simulink model "pi_SS_H2DF_2024a_GRU"  (R2024a)
settings: Solver=FixedStepAuto  StartTime=0.0  StopTime=inf  FixedStep=0.001  RelTol=1e-3  EnableMultiTasking=on
values from neighbouring files (symbols this model uses):
  C2C_NMPC = init_C2C_NMPC_H2DF(C2C_NMPC.expdata)    [run_SS_H2DF_control.m]
libraries: matrix_library x3, raspberrypiNetworklib x1
(part 1 of 3)
settings Model: SimulationMode=external  ExtModeTrigDuration=2  Creator=maxim  LastModifiedBy=winkler_a
settings SolverCC: PositivePriorityOrder=on
settings DataIOCC: LimitDataPoints=on  MaxDataPoints=10000  SaveOutput=off
settings OptimizationCC: EnhancedBackFolding=on  PassReuseOutputArgsAs=Individual arguments  ZeroExternalMemoryAtStartup=off  ZeroInternalMemoryAtStartup=off  MaxStackSize=64  OptimizeBlockOrder=speed  DifferentSizesBufferReuse=on  OptimizationCustomize=off  EfficientTunableParamExpr=on
settings DebuggingCC: ParameterTunabilityLossMsg=error
settings HardwareCC: ProdBitPerPointer=32  ProdBitPerSizeT=32  ProdBitPerPtrDiffT=32  ProdLargestAtomicInteger=Long  ProdLargestAtomicFloat=Double  ProdWordSize=32  ProdLongLongMode=on  ProdHWDeviceType=ARM Compatible->ARM Cortex
settings SFSimCC: SimUserSources=|
  | C2C_NMPC_model/C2C_NMPC_dyn_disc_phi_fun.c
  | C2C_NMPC_model/C2C_NMPC_dyn_disc_phi_fun_jac.c
  | C2C_NMPC_constraints/C2C_NMPC_constr_h_fun.c
  | C2C_NMPC_constraints/C2C_NMPC_constr_h_fun_jac_uxt_zt.c
  | C2C_NMPC_constraints/C2C_NMPC_constr_h_e_fun.c
  | C2C_NMPC_constraints/C2C_NMPC_constr_h_e_fun_jac_uxt_zt.c
  | acados_solver_sfunction_C2C_NMPC.c
  | acados_solver_C2C_NMPC.c
settings SFSimCC: SimUserIncludeDirs=|
  | /include
  | /include/acados_c
  | /include/blasfeo/include
  | /include/hpipm/include
  | /lib
  | /c_generated_code
settings SFSimCC: SimUserLibraries=|
  | libblasfeo.so
  | libacados.so
  | libhpipm.so
settings RTWCC: Description=Embedded Coder  SystemTargetFile=ert.tlc  HardwareBoard=Raspberry Pi  TemplateMakefile=ert_default_tmf  RTWUseSimCustomCode=on  Toolchain=GNU GCC Embedded Linux  BuildConfiguration=Faster Runs  GPUComputeCapability=3.5
settings RTWCC: CustomInclude=|
  | /include
  | /include/acados_c
  | /include/blasfeo/include
  | /include/hpipm/include
  | /lib
  | /c_generated_code
settings RTWCC: CustomSource=|
  | C2C_NMPC_model/C2C_NMPC_dyn_disc_phi_fun.c
  | C2C_NMPC_model/C2C_NMPC_dyn_disc_phi_fun_jac.c
  | C2C_NMPC_constraints/C2C_NMPC_constr_h_fun.c
  | C2C_NMPC_constraints/C2C_NMPC_constr_h_fun_jac_uxt_zt.c
  | C2C_NMPC_constraints/C2C_NMPC_constr_h_e_fun.c
  | C2C_NMPC_constraints/C2C_NMPC_constr_h_e_fun_jac_uxt_zt.c
  | acados_solver_sfunction_C2C_NMPC.c
  | acados_solver_C2C_NMPC.c
settings RTWCC: CustomLibrary=|
  | libblasfeo.so
  | libacados.so
  | libhpipm.so
settings CodeAppCC: ForceParamTrailComments=on  IgnoreCustomStorageClasses=off  OperatorAnnotations=on  SimulinkDataObjDesc=on  SFDataObjDesc=on  InsertBlockDesc=on
settings ERTTargetCC: SupportContinuousTime=on  SupportNonInlinedSFcns=on  SupportVariableSizeSignals=on  ExtMode=on  ExtModeStaticAlloc=on  ExtModeMaxTrigDuration=1000  ExtModeMexArgs='192.168.140.200' 0 17725

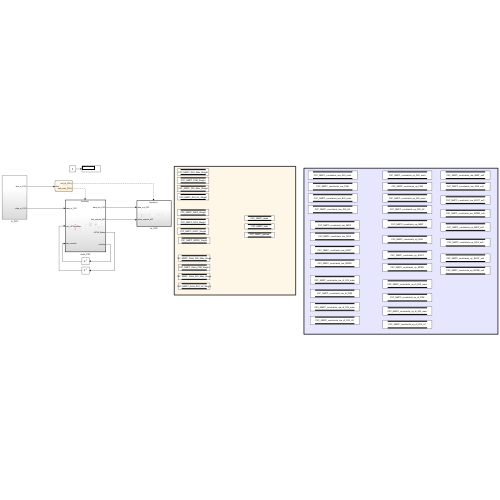
[thumbnail: Simulink's stored preview of the top-level diagram]
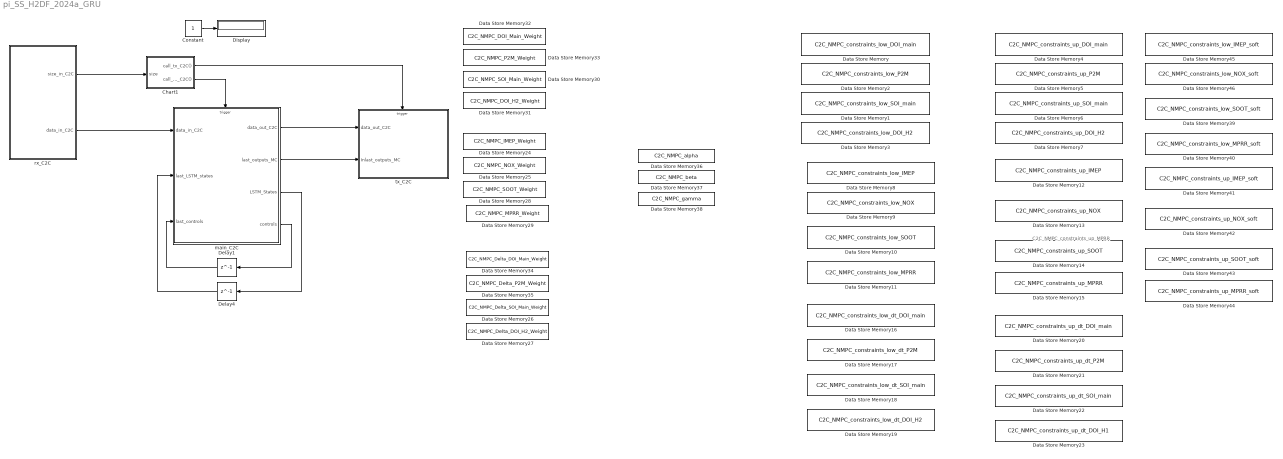
== system pi_SS_H2DF_2024a_GRU ==
  note: C2C_NMPC_constraints_up_MPRR
  Chart1 : Stateflow chart  TreatAsAtomicUnit=on
  Constant : Constant
  Data Store Memory : DataStoreMemory  DataStoreName=C2C_NMPC_constraints_low_DOI_main  WriteAfterWriteMsg=warning  ShowAdditionalParam=off
  Data Store Memory1 : DataStoreMemory  DataStoreName=C2C_NMPC_constraints_low_SOI_main  WriteAfterWriteMsg=warning  ShowAdditionalParam=off
  Data Store Memory10 : DataStoreMemory  DataStoreName=C2C_NMPC_constraints_low_SOOT  WriteAfterWriteMsg=warning  ShowAdditionalParam=off
  Data Store Memory11 : DataStoreMemory  DataStoreName=C2C_NMPC_constraints_low_MPRR  WriteAfterWriteMsg=warning  ShowAdditionalParam=off
  Data Store Memory12 : DataStoreMemory  DataStoreName=C2C_NMPC_constraints_up_IMEP  WriteAfterWriteMsg=warning  ShowAdditionalParam=off
  Data Store Memory13 : DataStoreMemory  DataStoreName=C2C_NMPC_constraints_up_NOX  WriteAfterWriteMsg=warning  ShowAdditionalParam=off
  Data Store Memory14 : DataStoreMemory  DataStoreName=C2C_NMPC_constraints_up_SOOT  WriteAfterWriteMsg=warning  ShowAdditionalParam=off
  Data Store Memory15 : DataStoreMemory  DataStoreName=C2C_NMPC_constraints_up_MPRR  WriteAfterWriteMsg=warning  ShowAdditionalParam=off
  Data Store Memory16 : DataStoreMemory  DataStoreName=C2C_NMPC_constraints_low_dt_DOI_main  WriteAfterWriteMsg=warning  ShowAdditionalParam=off
  Data Store Memory17 : DataStoreMemory  DataStoreName=C2C_NMPC_constraints_low_dt_P2M  WriteAfterWriteMsg=warning  ShowAdditionalParam=off
  Data Store Memory18 : DataStoreMemory  DataStoreName=C2C_NMPC_constraints_low_dt_SOI_main  WriteAfterWriteMsg=warning  ShowAdditionalParam=off
  Data Store Memory19 : DataStoreMemory  DataStoreName=C2C_NMPC_constraints_low_dt_DOI_H2  WriteAfterWriteMsg=warning  ShowAdditionalParam=off
  Data Store Memory2 : DataStoreMemory  DataStoreName=C2C_NMPC_constraints_low_P2M  WriteAfterWriteMsg=warning  ShowAdditionalParam=off
  Data Store Memory20 : DataStoreMemory  DataStoreName=C2C_NMPC_constraints_up_dt_DOI_main  WriteAfterWriteMsg=warning  ShowAdditionalParam=off
  Data Store Memory21 : DataStoreMemory  DataStoreName=C2C_NMPC_constraints_up_dt_P2M  WriteAfterWriteMsg=warning  ShowAdditionalParam=off
  Data Store Memory22 : DataStoreMemory  DataStoreName=C2C_NMPC_constraints_up_dt_SOI_main  WriteAfterWriteMsg=warning  ShowAdditionalParam=off
  Data Store Memory23 : DataStoreMemory  DataStoreName=C2C_NMPC_constraints_up_dt_DOI_H1  WriteAfterWriteMsg=warning  ShowAdditionalParam=off
  Data Store Memory24 : DataStoreMemory  DataStoreName=C2C_NMPC_IMEP_Weight  WriteAfterWriteMsg=warning  ShowAdditionalParam=off
  Data Store Memory25 : DataStoreMemory  DataStoreName=C2C_NMPC_NOX_Weight  WriteAfterWriteMsg=warning  ShowAdditionalParam=off
  Data Store Memory26 : DataStoreMemory  DataStoreName=C2C_NMPC_Delta_SOI_Main_Weight  WriteAfterWriteMsg=warning  ShowAdditionalParam=off
  Data Store Memory27 : DataStoreMemory  DataStoreName=C2C_NMPC_Delta_DOI_H2_Weight  WriteAfterWriteMsg=warning  ShowAdditionalParam=off
  Data Store Memory28 : DataStoreMemory  DataStoreName=C2C_NMPC_SOOT_Weight  WriteAfterWriteMsg=warning  ShowAdditionalParam=off
  Data Store Memory29 : DataStoreMemory  DataStoreName=C2C_NMPC_MPRR_Weight  WriteAfterWriteMsg=warning  ShowAdditionalParam=off
  Data Store Memory3 : DataStoreMemory  DataStoreName=C2C_NMPC_constraints_low_DOI_H2  WriteAfterWriteMsg=warning  ShowAdditionalParam=off
  Data Store Memory30 : DataStoreMemory  DataStoreName=C2C_NMPC_SOI_Main_Weight  WriteAfterWriteMsg=warning  ShowAdditionalParam=off
  Data Store Memory31 : DataStoreMemory  DataStoreName=C2C_NMPC_DOI_H2_Weight  WriteAfterWriteMsg=warning  ShowAdditionalParam=off
  Data Store Memory32 : DataStoreMemory  DataStoreName=C2C_NMPC_DOI_Main_Weight  WriteAfterWriteMsg=warning  ShowAdditionalParam=off
  Data Store Memory33 : DataStoreMemory  DataStoreName=C2C_NMPC_P2M_Weight  WriteAfterWriteMsg=warning  ShowAdditionalParam=off
  Data Store Memory34 : DataStoreMemory  DataStoreName=C2C_NMPC_Delta_DOI_Main_Weight  WriteAfterWriteMsg=warning  ShowAdditionalParam=off
  Data Store Memory35 : DataStoreMemory  DataStoreName=C2C_NMPC_Delta_P2M_Weight  WriteAfterWriteMsg=warning  ShowAdditionalParam=off
  Data Store Memory36 : DataStoreMemory  DataStoreName=C2C_NMPC_alpha  WriteAfterWriteMsg=warning  ShowAdditionalParam=off
  Data Store Memory37 : DataStoreMemory  DataStoreName=C2C_NMPC_beta  WriteAfterWriteMsg=warning  ShowAdditionalParam=off
  Data Store Memory38 : DataStoreMemory  DataStoreName=C2C_NMPC_gamma  WriteAfterWriteMsg=warning  ShowAdditionalParam=off
  Data Store Memory39 : DataStoreMemory  DataStoreName=C2C_NMPC_constraints_low_SOOT_soft  WriteAfterWriteMsg=warning  ShowAdditionalParam=off
  Data Store Memory4 : DataStoreMemory  DataStoreName=C2C_NMPC_constraints_up_DOI_main  WriteAfterWriteMsg=warning  ShowAdditionalParam=off
  Data Store Memory40 : DataStoreMemory  DataStoreName=C2C_NMPC_constraints_low_MPRR_soft  WriteAfterWriteMsg=warning  ShowAdditionalParam=off
  Data Store Memory41 : DataStoreMemory  DataStoreName=C2C_NMPC_constraints_up_IMEP_soft  WriteAfterWriteMsg=warning  ShowAdditionalParam=off
  Data Store Memory42 : DataStoreMemory  DataStoreName=C2C_NMPC_constraints_up_NOX_soft  WriteAfterWriteMsg=warning  ShowAdditionalParam=off
  Data Store Memory43 : DataStoreMemory  DataStoreName=C2C_NMPC_constraints_up_SOOT_soft  WriteAfterWriteMsg=warning  ShowAdditionalParam=off
  Data Store Memory44 : DataStoreMemory  DataStoreName=C2C_NMPC_constraints_up_MPRR_soft  WriteAfterWriteMsg=warning  ShowAdditionalParam=off
  Data Store Memory45 : DataStoreMemory  DataStoreName=C2C_NMPC_constraints_low_IMEP_soft  WriteAfterWriteMsg=warning  ShowAdditionalParam=off
  Data Store Memory46 : DataStoreMemory  DataStoreName=C2C_NMPC_constraints_low_NOX_soft  WriteAfterWriteMsg=warning  ShowAdditionalParam=off
  Data Store Memory5 : DataStoreMemory  DataStoreName=C2C_NMPC_constraints_up_P2M  WriteAfterWriteMsg=warning  ShowAdditionalParam=off
  Data Store Memory6 : DataStoreMemory  DataStoreName=C2C_NMPC_constraints_up_SOI_main  WriteAfterWriteMsg=warning  ShowAdditionalParam=off
  Data Store Memory7 : DataStoreMemory  DataStoreName=C2C_NMPC_constraints_up_DOI_H2  WriteAfterWriteMsg=warning  ShowAdditionalParam=off
  Data Store Memory8 : DataStoreMemory  DataStoreName=C2C_NMPC_constraints_low_IMEP  WriteAfterWriteMsg=warning  ShowAdditionalParam=off
  Data Store Memory9 : DataStoreMemory  DataStoreName=C2C_NMPC_constraints_low_NOX  WriteAfterWriteMsg=warning  ShowAdditionalParam=off
  Delay1 : Delay  DelayLength=1  InitialCondition=C2C_NMPC.x0([(C2C_NMPC.Dims.n_LSTM_states + 1):(C2C_NMPC.Dims.n_LSTM_states + C2C_NMPC.Dims.n_controls)])
  Delay4 : Delay  DelayLength=1  InitialCondition=C2C_NMPC.x0(1:C2C_NMPC.Dims.n_LSTM_states)
  Display : Display
  main_C2C : Subsystem
  rx_C2C : Subsystem
  tx_C2C : Subsystem
  wires:
  rx_C2C/1(size_in_C2C) -> Chart1/1(size)
  rx_C2C/2(data_in_C2C) -> main_C2C/1(data_in_C2C)
  Chart1/2(call_main_C2C()) -> main_C2C/Trigger
  Constant/1 -> Display/1
  main_C2C/1(data_out_C2C) -> tx_C2C/1(data_out_C2C)
  main_C2C/2(last_outputs_MC) -> tx_C2C/2(Inlast_outputs_MC)
  Chart1/1(call_tx_C2C()) -> tx_C2C/Trigger
  main_C2C/4(controls) -> Delay1/1
  main_C2C/3(LSTM_States) -> Delay4/1
  Delay1/1 -> main_C2C/3(last_controls)
  Delay4/1 -> main_C2C/2(last_LSTM_states)

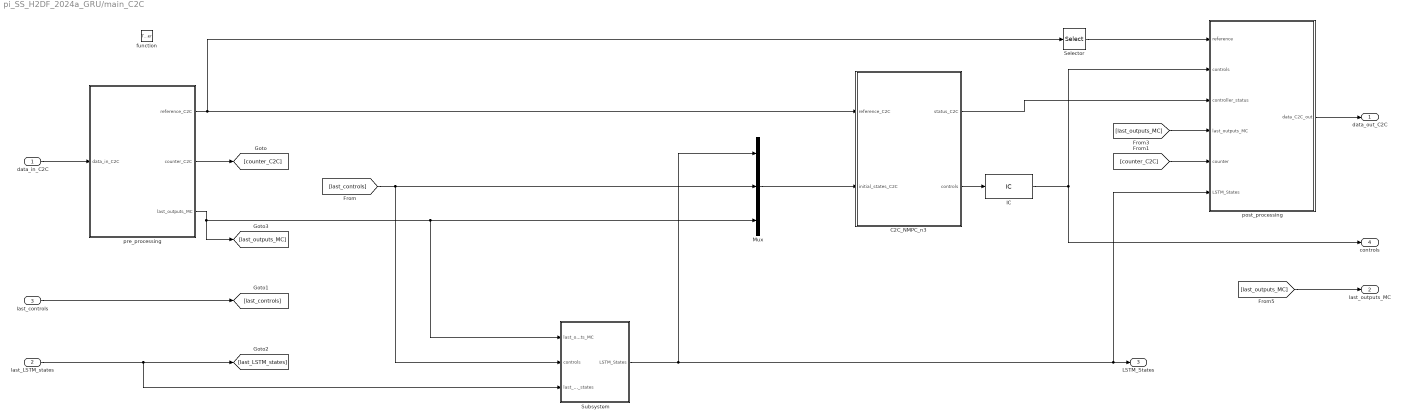
== system pi_SS_H2DF_2024a_GRU/main_C2C ==
  data_in_C2C : Inport
  last_LSTM_states : Inport  Port=2
  last_controls : Inport  Port=3
  function : TriggerPort  TriggerType=function-call  VariantControl=(inherit)
  C2C_NMPC_n3 : Subsystem  VariantControl=C2C_NMPC_n3
  IC : InitialCondition  Value=C2C_NMPC.x0([(C2C_NMPC.Dims.n_LSTM_states + 1):(C2C_NMPC.Dims.n_LSTM_states + C2C_NMPC.Dims.n_controls)])
  Mux : Mux  Inputs=3
  Selector : Selector  InputPortWidth=C2C_NMPC.Dims.n_cost*3  IndexOptions=Index vector (dialog)  Indices=1:C2C_NMPC.Dims.n_cost  OutputSizes=1
  Subsystem : Subsystem
  post_processing : Subsystem
  pre_processing : Subsystem
  data_out_C2C : Outport
  last_outputs_MC : Outport  Port=2
  LSTM_States : Outport  Port=3
  controls : Outport  Port=4
  wires:
  IC/1 -> post_processing/2(controls), controls/1
  C2C_NMPC_n3/2(controls) -> IC/1
  last_LSTM_states/1 -> Subsystem/3(last_LSTM_states), [last_LSTM_states]
  data_in_C2C/1 -> pre_processing/1(data_in_C2C)
  Subsystem/1(LSTM_States) -> Mux/1, post_processing/6(LSTM_States), LSTM_States/1
  Mux/1 -> C2C_NMPC_n3/2(initial_states_C2C)
  pre_processing/2(counter_C2C) -> [counter_C2C]
  pre_processing/3(last_outputs_MC) -> Subsystem/1(last_outputs_MC), Mux/3, [last_outputs_MC]
  [last_outputs_MC] -> last_outputs_MC/1
  [counter_C2C] -> post_processing/5(counter)
  Selector/1 -> post_processing/1(reference)
  last_controls/1 -> [last_controls]
  [last_outputs_MC] -> post_processing/4(last_outputs_MC)
  [last_controls] -> Subsystem/2(controls), Mux/2
  C2C_NMPC_n3/1(status_C2C) -> post_processing/3(controller_status)
  post_processing/1(data_C2C_out) -> data_out_C2C/1
  pre_processing/1(reference_C2C) -> C2C_NMPC_n3/1(reference_C2C), Selector/1

== system pi_SS_H2DF_2024a_GRU/rx_C2C ==
  Data Type Conversion : DataTypeConversion  OutDataTypeStr=double  SaturateOnIntegerOverflow=off  RndMeth=Floor
  Receive : Subsystem
  Terminator : Terminator
  UDP Receive1 : raspberrypiNetworklib/UDP Receive  localURL='0.0.0.0'  localPort=42785  remoteURL='0.0.0.0'  remotePort=-1  recvBufferSize=8192  signalDatatype=uint32  dims=56  isVarSize=off  showBlockingTime=off  blockingTime=0  sampletime=0.001  blockPlatform=Raspberry Pi
  size_in_C2C : Outport
  data_in_C2C : Outport  Port=2
  wires:
  UDP Receive1/2 -> size_in_C2C/1
  UDP Receive1/1 -> Data Type Conversion/1
  Receive/1(udp_outputs) -> data_in_C2C/1
  Data Type Conversion/1 -> Receive/1(udp_data_in)
  Receive/2(controller_mode) -> Terminator/1

== system pi_SS_H2DF_2024a_GRU/tx_C2C ==
  note: [1:4,13,99:134,14,15,16,17,71:74]
  data_out_C2C : Inport
  Inlast_outputs_MC : Inport  Port=2
  function : TriggerPort  TriggerType=function-call  VariantControl=(inherit)
  Data Type Conversion : DataTypeConversion  OutDataTypeStr=uint32  SaturateOnIntegerOverflow=off  RndMeth=Floor
  Selector : Selector  IndexOptions=Index vector (dialog)  Indices=[1:4,13,115:142,14,15,16,17,95:98]  OutputSizes=1
  Subsystem : Subsystem
  Terminator : Terminator
  UDP Send1 : S-Function  AncestorBlock=raspberrypiNetworklib/UDP Send  InitFcn=|  FunctionName=sdspToNetwork  Parameters=localURL, localPortSource, localPort, remoteURL, remotePort, 8192, separateLengthPort, []  SFunctionDeploymentMode=off  EnableBusSupport=off  mask(UDP Send){remoteURL='192.168.140.159', remotePort=42784, localURL='0.0.0.0', localPortSource=Specify via dialog, localPort=42784, sampletime=-1, blockPlatform=Raspberry Pi, separateLengthPort=0}
      | realtime.internal.validateLinuxBlock(get_param(gcbh, 'blockPlatform'), gcbh);
      | realtime.internal.registerLinuxBlock(gcb);
      mask prompts: remoteURL "Remote IP address ('255.255.255.255' for broadcast):"; remotePort "Remote IP port:"; localURL "Local IP address:"; localPortSource "Local IP port source:"; localPort "Local IP port:"; blockPlatform "Block Platform"; separateLengthPort "Use a separate length port"
      mask help: Sends UDP packets to another UDP host on an Internet network. Set Remote IP address parameter to the IP address of the receiving UDP host. Set the Remote IP port parameter to the port number used by the receiving UDP host.
      mask Help: eval('realtime.helpView(get_param(gcb, ''blockPlatform''), [realtime.internal.getHelpLinkPrefix(gcb) ''libudpsend''])');
      mask TypeOptions localPortSource: Automatically determine | Specify via dialog
      mask Callback localPortSource:
      | mask_vis = get_param(gcbh, 'MaskVisibilities');
      | if strcmp(get_param(gcbh,'localPortSource'),'Specify via dialog')
      |     mask_vis{5} = 'on';
      | else
      |     mask_vis{5} = 'off';
      | end
      | set_param(gcbh, 'MaskVisibilities', mask_vis);
      | clear('mask_vis');
      mask Display:
      | %fprintf('UDP Send');
      | color('blue');
      | [data, map]=imread('ethernet2_bw.gif');pic=ind2rgb(data,map);image(pic,[0.32 0.25 0.40 0.45]);
      | platform = realtime.internal.getBlockDisplayText(gcb);
      | text(0.99, 0.9, platform, 'horizontalalignment', 'right');
  wires:
  data_out_C2C/1 -> Selector/1
  Data Type Conversion/1 -> UDP Send1/1
  Selector/1 -> Subsystem/1(In1)
  Subsystem/1(Out1) -> Data Type Conversion/1
  Inlast_outputs_MC/1 -> Terminator/1

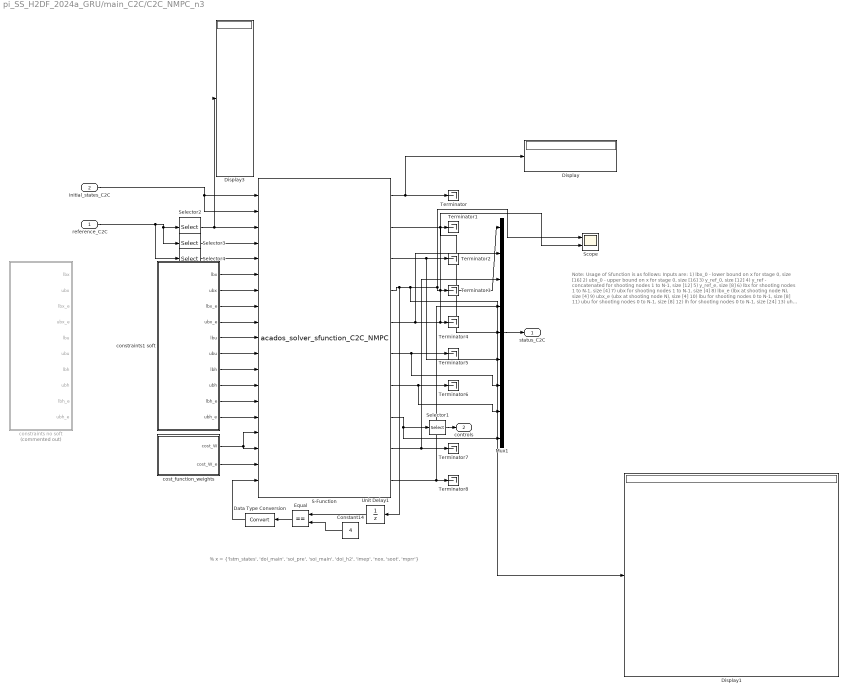
== system pi_SS_H2DF_2024a_GRU/main_C2C/C2C_NMPC_n3 ==
  note: Note: Usage of Sfunction is as follows:
      | Inputs are:
      | 1) lbx_0 - lower bound on x for stage 0, size [16]
      | 2) ubx_0 - upper bound on x for stage 0, size [16]
      | 3) y_ref_0, size [12]
      | 4) y_ref - concatenated for shooting nodes 1 to N-1, size [12]
      | 5) y_ref_e, size [8]
      | 6) lbx for shooting nodes 1 to N-1, size [4]
      | 7) ubx for shooting nodes 1 to N-1, size [4]
      | 8) lbx_e (lbx at shooting node N), size [4]
      | 9) ubx_e (ubx at shooting node N), size [4]
      | 10) lbu for shooting nodes 0 to N-1, size [8]
      | 11) ubu for shooting nodes 0 to N-1, size [8]
      | 12) lh for shooting nodes 0 to N-1, size [24]
      | 13) uh for shooting nodes 0 to N-1, size [24]
      | 14) lh_e, size [8]
      | 15) uh_e, size [8]
      | 16) cost_W_0 in column-major format, size [144]
      | 17) cost_W in column-major format, that is set for all intermediate shooting nodes: 1 to N-1, size [144]
      | 18) cost_W_e in column-major format, size [64]
      | 19) reset_solver determines if iterate is set to all zeros before other initializations (x_init, u_init) are set and before solver is called, size [1]
      |
      | Outputs are:
      | 1) u0, control input at node 0, size [4]
      | 2) utraj, control input concatenated for nodes 0 to N-1, size [8]
      | 3) xtraj, state concatenated for nodes 0 to N, size [48]
      | 4) acados solver status (0 = SUCCESS)
      | 5) cost function value
      | 6) KKT residual
      | 7) KKT residuals, size [4] (stat, eq, ineq, comp)
      | 8) x1, state at node 1
      | 9) CPU time
      | 10) SQP iterations
  note: % x = {'lstm_states', 'doi_main', 'soi_pre', 'soi_main', 'doi_h2', 'imep', 'nox, 'soot', 'mprr'}
  reference_C2C : Inport
  initial_states_C2C : Inport  Port=2
  Constant14 : Constant  Value=4
  Data Type Conversion : DataTypeConversion  SaturateOnIntegerOverflow=off  RndMeth=Floor
  Display : Display
  Display1 : Display
  Display3 : Display
  Equal : RelationalOperator  Operator===  OutDataTypeStr=boolean  RndMeth=Simplest  InputSameDT=off
  Mux1 : Mux  Inputs=9
  S-Function : S-Function  FunctionName=acados_solver_sfunction_C2C_NMPC  SFunctionDeploymentMode=off  EnableBusSupport=off
  Scope : Scope  NumInputPorts=2
  Selector1 : Selector  IndexOptions=Index vector (dialog)  Indices=[(C2C_NMPC.Dims.n_LSTM_states + 1):(C2C_NMPC.Dims.n_LSTM_states + C2C_NMPC.Dims.n_controls)]  OutputSizes=1
  Selector2 : Selector  IndexOptions=Index vector (dialog)  Indices=[1:(C2C_NMPC.Dims.n_cost)]  OutputSizes=1
  Selector3 : Selector  IndexOptions=Index vector (dialog)  Indices=[ (C2C_NMPC.Dims.n_cost + 1) : (C2C_NMPC.Dims.n_cost * 3) ]  OutputSizes=1
  Selector4 : Selector  IndexOptions=Index vector (dialog)  Indices=[ (C2C_NMPC.Dims.n_cost * 2 + 1) : (C2C_NMPC.Dims.n_cost * 2 + C2C_NMPC.Dims.n_controls + C2C_NMPC.Dims.n_outputs ) ]  OutputSizes=1
  Terminator{,1..8} (9 alike) : Terminator
  Unit Delay1 : UnitDelay  SampleTime=-1  HasFrameUpgradeWarning=on
  constraints no soft : Subsystem  Commented=on
  "constraints1 soft " : Subsystem
  cost_function_weights : Subsystem
  status_C2C : Outport
  controls : Outport  Port=2
  wires:
  "constraints1 soft "/5(lbu) -> S-Function/10
  "constraints1 soft "/6(ubu) -> S-Function/11
  "constraints1 soft "/7(lbh) -> S-Function/12
  "constraints1 soft "/8(ubh) -> S-Function/13
  "constraints1 soft "/9(lbh_e) -> S-Function/14
  "constraints1 soft "/10(ubh_e) -> S-Function/15
  cost_function_weights/1(cost_W) -> S-Function/16, S-Function/17
  Data Type Conversion/1 -> S-Function/19
  cost_function_weights/2(cost_W_e) -> S-Function/18
  "constraints1 soft "/1(lbx) -> S-Function/6
  "constraints1 soft "/2(ubx) -> S-Function/7
  "constraints1 soft "/3(lbx_e) -> S-Function/8
  "constraints1 soft "/4(ubx_e) -> S-Function/9
  S-Function/5 -> Mux1/2, Terminator4/1, Scope/2
  Equal/1 -> Data Type Conversion/1
  Unit Delay1/1 -> Equal/1
  Constant14/1 -> Equal/2
  Mux1/1 -> status_C2C/1
  Selector1/1 -> controls/1
  Selector4/1 -> S-Function/5
  reference_C2C/1 -> Selector4/1, Selector3/1, Selector2/1
  initial_states_C2C/1 -> S-Function/1, S-Function/2
  S-Function/10 -> Terminator8/1, Mux1/4
  S-Function/9 -> Terminator7/1, Mux1/3
  S-Function/7 -> Terminator6/1, Mux1/8
  S-Function/6 -> Terminator5/1, Mux1/7
  S-Function/8 -> Selector1/1, Mux1/9
  S-Function/4 -> Unit Delay1/1, Scope/1, Mux1/1, Terminator3/1, Display1/1
  S-Function/3 -> Terminator2/1, Mux1/6
  S-Function/2 -> Terminator1/1, Mux1/5
  S-Function/1 -> Display/1, Terminator/1
  Selector2/1 -> Display3/1, S-Function/3
  Selector3/1 -> S-Function/4

== system pi_SS_H2DF_2024a_GRU/main_C2C/Subsystem ==
  last_outputs_MC : Inport
  controls : Inport  Port=2
  last_LSTM_states : Inport  Port=3
  dyn_H2DF_state_augmentation : Subsystem
  LSTM_States : Outport
  wires:
  dyn_H2DF_state_augmentation/1(LSTM_states) -> LSTM_States/1
  controls/1 -> dyn_H2DF_state_augmentation/2(controls)
  last_outputs_MC/1 -> dyn_H2DF_state_augmentation/1(last_outputs_MC)
  last_LSTM_states/1 -> dyn_H2DF_state_augmentation/3(last_LSTM_states)

== system pi_SS_H2DF_2024a_GRU/main_C2C/post_processing ==
  reference : Inport
  controls : Inport  Port=2
  controller_status : Inport  Port=3
  last_outputs_MC : Inport  Port=4
  counter : Inport  Port=5
  LSTM_States : Inport  Port=6
  " denormalizing reference" : Subsystem
  Demux1 : Demux
  Demux2 : Demux
  Demux3 : Demux
  Display : Display  Commented=on
  Mux{8..11} (4 alike) : Mux  Inputs=2
  Mux4 : Mux
  Mux5 : Mux  Inputs=6
  Mux6 : Mux
  Selector5 : Selector  IndexOptions=Index vector (dialog)  Indices=[(C2C_NMPC.Dims.n_controls + 1 ):(C2C_NMPC.Dims.n_cost - C2C_NMPC.Dims.n_controls)]  OutputSizes=1
  Subsystem1 : Subsystem
  denormalizing physical controls and outputs : Subsystem
  data_C2C_out : Outport
  wires:
  Demux3/1 -> " denormalizing reference"/1(IMEP_norm)
  Demux3/2 -> " denormalizing reference"/2(NOX_norm)
  Demux3/4 -> " denormalizing reference"/4(MPRR_norm)
  Demux3/3 -> " denormalizing reference"/3(soot_norm)
  reference/1 -> Selector5/1
  Selector5/1 -> Demux3/1
  controls/1 -> Demux2/1
  Demux1/1 -> denormalizing physical controls and outputs/1(IMEP_norm)
  Demux1/2 -> denormalizing physical controls and outputs/2(NOX_norm)
  Demux1/3 -> denormalizing physical controls and outputs/3(soot_norm)
  Demux1/4 -> denormalizing physical controls and outputs/4(MPRR_norm)
  Demux2/1 -> denormalizing physical controls and outputs/5(DOI_main_norm)
  Demux2/2 -> denormalizing physical controls and outputs/6(SOI_pre_norm)
  Demux2/3 -> denormalizing physical controls and outputs/7(SOI_main_norm)
  denormalizing physical controls and outputs/5(DOI_main) -> Mux6/1
  denormalizing physical controls and outputs/6(SOI_pre) -> Mux6/2
  denormalizing physical controls and outputs/7(SOI_main) -> Mux6/3
  " denormalizing reference"/1(IMEP) -> Mux11/1
  " denormalizing reference"/2(NOX) -> Mux9/1
  " denormalizing reference"/3(soot) -> Mux8/1
  " denormalizing reference"/4(MPRR) -> Mux10/1
  controller_status/1 -> Mux5/4, Subsystem1/1(controller_ status)
  Mux5/1 -> data_C2C_out/1
  Mux11/1 -> Mux4/1
  Mux8/1 -> Mux4/3
  Mux10/1 -> Mux4/4
  denormalizing physical controls and outputs/1(IMEP) -> Mux11/2
  denormalizing physical controls and outputs/2(NOX) -> Mux9/2
  denormalizing physical controls and outputs/3(soot) -> Mux8/2
  denormalizing physical controls and outputs/4(MPRR) -> Mux10/2
  Mux4/1 -> Mux5/2
  counter/1 -> Mux5/3
  Mux6/1 -> Display/1, Mux5/1
  Demux2/4 -> denormalizing physical controls and outputs/8(DOI_H2_norm)
  denormalizing physical controls and outputs/8(DOI_H2) -> Mux6/4
  Mux9/1 -> Mux4/2
  LSTM_States/1 -> Mux5/5
  last_outputs_MC/1 -> Subsystem1/2(Last_Output_MC), Demux1/1
  Subsystem1/1(Out1) -> Mux5/6

== system pi_SS_H2DF_2024a_GRU/main_C2C/pre_processing ==
  data_in_C2C : Inport
  Selector : Selector  IndexOptions=Index vector (dialog)  Indices=[6]  OutputSizes=1
  normalize_last_outputs_MC : Subsystem
  normalize_reference_C2C : Subsystem
  reference_C2C : Outport  VectorParamsAs1DForOutWhenUnconnected=off
  counter_C2C : Outport  Port=2  VectorParamsAs1DForOutWhenUnconnected=off
  last_outputs_MC : Outport  Port=3  VectorParamsAs1DForOutWhenUnconnected=off
  wires:
  normalize_reference_C2C/1(reference_C2C) -> reference_C2C/1
  data_in_C2C/1 -> Selector/1, normalize_last_outputs_MC/1(data_in), normalize_reference_C2C/1(data_in)
  normalize_last_outputs_MC/1(last_outputs_MC) -> last_outputs_MC/1
  Selector/1 -> counter_C2C/1

== system pi_SS_H2DF_2024a_GRU/rx_C2C/Receive ==
  note: block for horizon of 3 from engine
  udp_data_in : Inport
  conversion_n3 : Subsystem
  udp_outputs : Outport
  controller_mode : Outport  Port=2
  wires:
  udp_data_in/1 -> conversion_n3/1(udp_data_in)
  conversion_n3/1(udp_outputs) -> udp_outputs/1
  conversion_n3/2(controller_mode) -> controller_mode/1

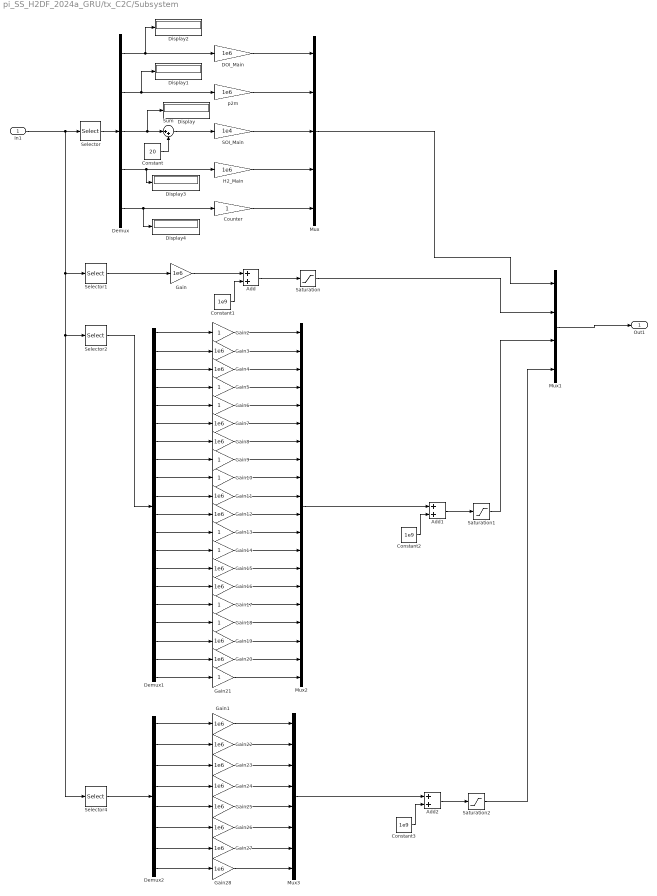
== system pi_SS_H2DF_2024a_GRU/tx_C2C/Subsystem ==
  In1 : Inport
  Add : Sum
  Add1 : Sum
  Add2 : Sum
  Constant : Constant  Value=20
  Constant1 : Constant  Value=1e9
  Constant2 : Constant  Value=1e9
  Constant3 : Constant  Value=1e9
  Counter : Gain
  DOI_Main : Gain  Gain=1e6
  Demux : Demux  Outputs=5
  Demux1 : Demux  Outputs=20
  Demux2 : Demux  Outputs=8
  Display{,1..4} (5 alike) : Display
  Gain{,1,3..4,7..8,11..12,15..16,19..20,22..28} (19 alike) : Gain  Gain=1e6
  Gain{2,5..6,9..10,13..14,17..18,21} (10 alike) : Gain
  H2_Main : Gain  Gain=1e6
  Mux : Mux  Inputs=5
  Mux1 : Mux
  Mux2 : Mux  Inputs=20
  Mux3 : Mux  Inputs=8
  SOI_Main : Gain  Gain=1e4
  Saturation : Saturate  UpperLimit=4e9  LowerLimit=0
  Saturation1 : Saturate  UpperLimit=4e9  LowerLimit=0
  Saturation2 : Saturate  UpperLimit=4e9  LowerLimit=0
  Selector : Selector  IndexOptions=Index vector (dialog)  Indices=[1:5]  OutputSizes=1
  Selector1 : Selector  IndexOptions=Index vector (dialog)  Indices=[6:13]  OutputSizes=1
  Selector2 : Selector  IndexOptions=Index vector (dialog)  Indices=[14:33]  OutputSizes=1
  Selector4 : Selector  IndexOptions=Index vector (dialog)  Indices=[34:41]  OutputSizes=1
  Sum : Sum  Inputs=|++
  p2m : Gain  Gain=1e6
  Out1 : Outport
  wires:
  Counter/1 -> Mux/5
  DOI_Main/1 -> Mux/1
  H2_Main/1 -> Mux/4
  SOI_Main/1 -> Mux/3
  In1/1 -> Selector4/1, Selector2/1, Selector1/1, Selector/1
  p2m/1 -> Mux/2
  Demux/1 -> Display2/1, DOI_Main/1
  Demux/2 -> Display1/1, p2m/1
  Demux/4 -> Display3/1, H2_Main/1
  Demux/5 -> Display4/1, Counter/1
  Demux/3 -> Display/1, Sum/1
  Sum/1 -> SOI_Main/1
  Constant/1 -> Sum/2
  Selector/1 -> Demux/1
  Gain/1 -> Add/1
  Constant1/1 -> Add/2
  Selector1/1 -> Gain/1
  Mux/1 -> Mux1/1
  Mux1/1 -> Out1/1
  Add/1 -> Saturation/1
  Saturation/1 -> Mux1/2
  Saturation1/1 -> Mux1/3
  Mux2/1 -> Add1/1
  Constant2/1 -> Add1/2
  Add1/1 -> Saturation1/1
  Selector2/1 -> Demux1/1
  Demux1/1 -> Gain2/1
  Demux1/2 -> Gain3/1
  Demux1/3 -> Gain4/1
  Demux1/4 -> Gain5/1
  Demux1/5 -> Gain6/1
  Demux1/6 -> Gain7/1
  Demux1/7 -> Gain8/1
  Demux1/8 -> Gain9/1
  Demux1/9 -> Gain10/1
  Demux1/10 -> Gain11/1
  Demux1/11 -> Gain12/1
  Demux1/12 -> Gain13/1
  Demux1/13 -> Gain14/1
  Demux1/14 -> Gain15/1
  Demux1/15 -> Gain16/1
  Demux1/16 -> Gain17/1
  Demux1/17 -> Gain18/1
  Demux1/18 -> Gain19/1
  Demux1/19 -> Gain20/1
  Demux1/20 -> Gain21/1
  Gain2/1 -> Mux2/1
  Gain3/1 -> Mux2/2
  Gain4/1 -> Mux2/3
  Gain5/1 -> Mux2/4
  Gain6/1 -> Mux2/5
  Gain7/1 -> Mux2/6
  Gain8/1 -> Mux2/7
  Gain9/1 -> Mux2/8
  Gain10/1 -> Mux2/9
  Gain11/1 -> Mux2/10
  Gain12/1 -> Mux2/11
  Gain13/1 -> Mux2/12
  Gain14/1 -> Mux2/13
  Gain16/1 -> Mux2/15
  Gain15/1 -> Mux2/14
  Gain17/1 -> Mux2/16
  Gain18/1 -> Mux2/17
  Gain19/1 -> Mux2/18
  Gain20/1 -> Mux2/19
  Gain21/1 -> Mux2/20
  Selector4/1 -> Demux2/1
  Demux2/1 -> Gain1/1
  Demux2/2 -> Gain22/1
  Demux2/3 -> Gain23/1
  Demux2/4 -> Gain24/1
  Gain1/1 -> Mux3/1
  Gain22/1 -> Mux3/2
  Gain23/1 -> Mux3/3
  Gain24/1 -> Mux3/4
  Saturation2/1 -> Mux1/4
  Mux3/1 -> Add2/1
  Constant3/1 -> Add2/2
  Add2/1 -> Saturation2/1
  Demux2/5 -> Gain25/1
  Demux2/6 -> Gain26/1
  Demux2/7 -> Gain27/1
  Demux2/8 -> Gain28/1
  Gain25/1 -> Mux3/5
  Gain26/1 -> Mux3/6
  Gain27/1 -> Mux3/7
  Gain28/1 -> Mux3/8

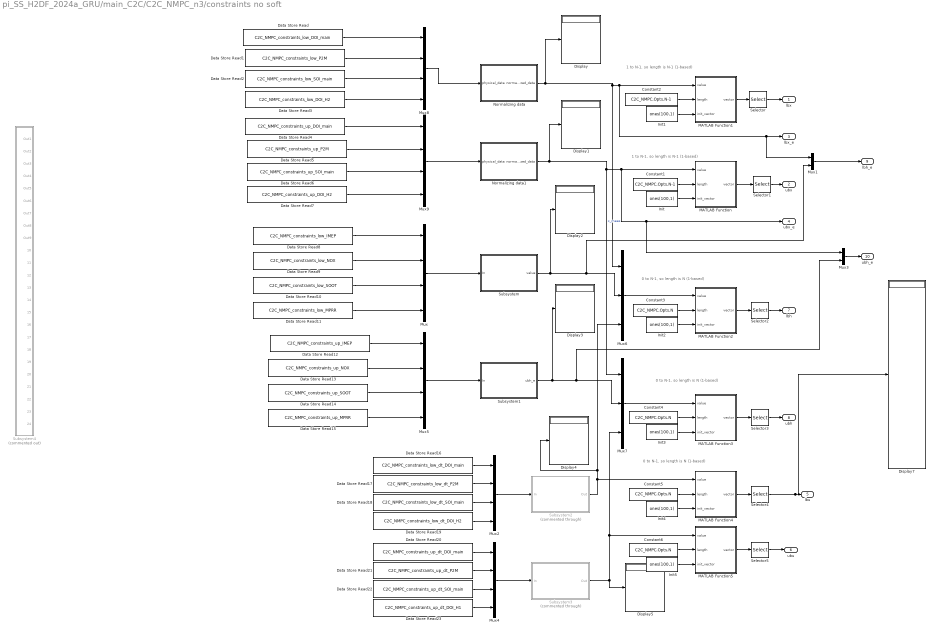
== system pi_SS_H2DF_2024a_GRU/main_C2C/C2C_NMPC_n3/constraints no soft ==
  note: 1 to N-1, so length is N-1 (1-based)
  note: 1 to N-1, so length is N-1 (1-based)
  note: 0 to N-1, so length is N (1-based)
  note: 0 to N-1, so length is N (1-based)
  note: 0 to N-1, so length is N (1-based)
  Constant1 : Constant  Value=C2C_NMPC.Opts.N-1
  Constant2 : Constant  Value=C2C_NMPC.Opts.N-1
  Constant{3..6} (4 alike) : Constant  Value=C2C_NMPC.Opts.N
  Data Store Read : DataStoreRead  DataStoreName=C2C_NMPC_constraints_low_DOI_main  IndexOptions=Index vector (dialog)  Indices=1  OutputSizes=1
  Data Store Read1 : DataStoreRead  DataStoreName=C2C_NMPC_constraints_low_P2M  IndexOptions=Index vector (dialog)  Indices=1  OutputSizes=1
  Data Store Read10 : DataStoreRead  DataStoreName=C2C_NMPC_constraints_low_SOOT  IndexOptions=Index vector (dialog)  Indices=1  OutputSizes=1
  Data Store Read11 : DataStoreRead  DataStoreName=C2C_NMPC_constraints_low_MPRR  IndexOptions=Index vector (dialog)  Indices=1  OutputSizes=1
  Data Store Read12 : DataStoreRead  DataStoreName=C2C_NMPC_constraints_up_IMEP  IndexOptions=Index vector (dialog)  Indices=1  OutputSizes=1
  Data Store Read13 : DataStoreRead  DataStoreName=C2C_NMPC_constraints_up_NOX  IndexOptions=Index vector (dialog)  Indices=1  OutputSizes=1
  Data Store Read14 : DataStoreRead  DataStoreName=C2C_NMPC_constraints_up_SOOT  IndexOptions=Index vector (dialog)  Indices=1  OutputSizes=1
  Data Store Read15 : DataStoreRead  DataStoreName=C2C_NMPC_constraints_up_MPRR  IndexOptions=Index vector (dialog)  Indices=1  OutputSizes=1
  Data Store Read16 : DataStoreRead  DataStoreName=C2C_NMPC_constraints_low_dt_DOI_main  IndexOptions=Index vector (dialog)  Indices=1  OutputSizes=1
  Data Store Read17 : DataStoreRead  DataStoreName=C2C_NMPC_constraints_low_dt_P2M  IndexOptions=Index vector (dialog)  Indices=1  OutputSizes=1
  Data Store Read18 : DataStoreRead  DataStoreName=C2C_NMPC_constraints_low_dt_SOI_main  IndexOptions=Index vector (dialog)  Indices=1  OutputSizes=1
  Data Store Read19 : DataStoreRead  DataStoreName=C2C_NMPC_constraints_low_dt_DOI_H2  IndexOptions=Index vector (dialog)  Indices=1  OutputSizes=1
  Data Store Read2 : DataStoreRead  DataStoreName=C2C_NMPC_constraints_low_SOI_main  IndexOptions=Index vector (dialog)  Indices=1  OutputSizes=1
  Data Store Read20 : DataStoreRead  DataStoreName=C2C_NMPC_constraints_up_dt_DOI_main  IndexOptions=Index vector (dialog)  Indices=1  OutputSizes=1
  Data Store Read21 : DataStoreRead  DataStoreName=C2C_NMPC_constraints_up_dt_P2M  IndexOptions=Index vector (dialog)  Indices=1  OutputSizes=1
  Data Store Read22 : DataStoreRead  DataStoreName=C2C_NMPC_constraints_up_dt_SOI_main  IndexOptions=Index vector (dialog)  Indices=1  OutputSizes=1
  Data Store Read23 : DataStoreRead  DataStoreName=C2C_NMPC_constraints_up_dt_DOI_H1  IndexOptions=Index vector (dialog)  Indices=1  OutputSizes=1
  Data Store Read3 : DataStoreRead  DataStoreName=C2C_NMPC_constraints_low_DOI_H2  IndexOptions=Index vector (dialog)  Indices=1  OutputSizes=1
  Data Store Read4 : DataStoreRead  DataStoreName=C2C_NMPC_constraints_up_DOI_main  IndexOptions=Index vector (dialog)  Indices=1  OutputSizes=1
  Data Store Read5 : DataStoreRead  DataStoreName=C2C_NMPC_constraints_up_P2M  IndexOptions=Index vector (dialog)  Indices=1  OutputSizes=1
  Data Store Read6 : DataStoreRead  DataStoreName=C2C_NMPC_constraints_up_SOI_main  IndexOptions=Index vector (dialog)  Indices=1  OutputSizes=1
  Data Store Read7 : DataStoreRead  DataStoreName=C2C_NMPC_constraints_up_DOI_H2  IndexOptions=Index vector (dialog)  Indices=1  OutputSizes=1
  Data Store Read8 : DataStoreRead  DataStoreName=C2C_NMPC_constraints_low_IMEP  IndexOptions=Index vector (dialog)  Indices=1  OutputSizes=1
  Data Store Read9 : DataStoreRead  DataStoreName=C2C_NMPC_constraints_low_NOX  IndexOptions=Index vector (dialog)  Indices=1  OutputSizes=1
  Display{,1..5,7} (7 alike) : Display
  Init{,1..5} (6 alike) : Constant  Value=ones(100,1)
  MATLAB Function : MATLAB Function  TreatAsAtomicUnit=on
  MATLAB Function1 : MATLAB Function  TreatAsAtomicUnit=on
  MATLAB Function2 : MATLAB Function  TreatAsAtomicUnit=on
  MATLAB Function3 : MATLAB Function  TreatAsAtomicUnit=on
  MATLAB Function4 : MATLAB Function  TreatAsAtomicUnit=on
  MATLAB Function5 : MATLAB Function  TreatAsAtomicUnit=on
  Mux{,2,4..5,8..9} (6 alike) : Mux
  Mux1 : Mux  Inputs=2
  Mux3 : Mux  Inputs=2
  Mux6 : Mux  Inputs=3
  Mux7 : Mux  Inputs=3
  Normalizing data : Subsystem
  Normalizing data1 : Subsystem
  Selector : Selector  IndexOptions=Index vector (dialog)  Indices=1:((C2C_NMPC.Opts.N-1)*C2C_NMPC.Dims.n_controls)  OutputSizes=1
  Selector1 : Selector  IndexOptions=Index vector (dialog)  Indices=1:((C2C_NMPC.Opts.N-1)*C2C_NMPC.Dims.n_controls)  OutputSizes=1
  Selector2 : Selector  IndexOptions=Index vector (dialog)  Indices=1:((C2C_NMPC.Opts.N)*(C2C_NMPC.Dims.n_outputs + C2C_NMPC.Dims.n_controls +C2C_NMPC.Dims.n_controls))  OutputSizes=1
  Selector3 : Selector  IndexOptions=Index vector (dialog)  Indices=1:((C2C_NMPC.Opts.N)*(C2C_NMPC.Dims.n_outputs + C2C_NMPC.Dims.n_controls +C2C_NMPC.Dims.n_controls))  OutputSizes=1
  Selector4 : Selector  IndexOptions=Index vector (dialog)  Indices=1:((C2C_NMPC.Opts.N)*(C2C_NMPC.Dims.n_controls))  OutputSizes=1
  Selector5 : Selector  IndexOptions=Index vector (dialog)  Indices=1:((C2C_NMPC.Opts.N)*(C2C_NMPC.Dims.n_controls))  OutputSizes=1
  Subsystem : Subsystem
  Subsystem1 : Subsystem
  Subsystem2 : Subsystem  Commented=through
  Subsystem3 : Subsystem  Commented=through
  Subsystem4 : Subsystem  Commented=on
  lbx : Outport
  ubx : Outport  Port=2
  lbx_e : Outport  Port=3
  ubx_e : Outport  Port=4
  lbu : Outport  Port=5
  ubu : Outport  Port=6
  lbh : Outport  Port=7
  ubh : Outport  Port=8
  lbh_e : Outport  Port=9
  ubh_e : Outport  Port=10
  wires:
  Selector4/1 -> lbu/1, Display7/1
  Selector5/1 -> ubu/1
  Constant6/1 -> MATLAB Function5/2(length)
  Init5/1 -> MATLAB Function5/3(init_vector)
  MATLAB Function5/1(vector) -> Selector5/1
  MATLAB Function4/1(vector) -> Selector4/1
  Init4/1 -> MATLAB Function4/3(init_vector)
  Constant5/1 -> MATLAB Function4/2(length)
  Data Store Read23/1 -> Mux4/4
  Data Store Read22/1 -> Mux4/3
  Data Store Read21/1 -> Mux4/2
  Data Store Read20/1 -> Mux4/1
  Data Store Read19/1 -> Mux2/4
  Data Store Read18/1 -> Mux2/3
  Data Store Read17/1 -> Mux2/2
  Data Store Read16/1 -> Mux2/1
  Data Store Read15/1 -> Mux5/4
  Data Store Read14/1 -> Mux5/3
  Data Store Read13/1 -> Mux5/2
  Data Store Read12/1 -> Mux5/1
  Data Store Read11/1 -> Mux/4
  Data Store Read10/1 -> Mux/3
  Data Store Read9/1 -> Mux/2
  Data Store Read8/1 -> Mux/1
  Mux3/1 -> ubh_e/1
  Subsystem1/1(ubh_e) -> Mux7/2, Mux3/2, Display3/1
  Mux1/1 -> lbh_e/1
  Selector3/1 -> ubh/1
  Selector2/1 -> lbh/1
  Selector1/1 -> ubx/1
  Data Store Read7/1 -> Mux9/4
  Normalizing data1/1(normalized_data) -> MATLAB Function/1(value), ubx_e/1, Mux3/1, Mux7/1, Display1/1  "x_meas"
  Mux9/1 -> Normalizing data1/1(physical_data)
  Data Store Read4/1 -> Mux9/1
  Data Store Read5/1 -> Mux9/2
  Data Store Read6/1 -> Mux9/3
  Selector/1 -> lbx/1
  Mux8/1 -> Normalizing data/1(physical_data)
  Data Store Read/1 -> Mux8/1
  Data Store Read1/1 -> Mux8/2
  Data Store Read2/1 -> Mux8/3
  Data Store Read3/1 -> Mux8/4
  Constant4/1 -> MATLAB Function3/2(length)
  Init3/1 -> MATLAB Function3/3(init_vector)
  Mux7/1 -> MATLAB Function3/1(value)
  MATLAB Function3/1(vector) -> Selector3/1
  Subsystem2/1(Out) -> Mux6/3, Display4/1, MATLAB Function4/1(value)
  Subsystem/1(value) -> Mux6/2, Mux1/2, Display2/1
  Normalizing data/1(normalized_data) -> Display/1, MATLAB Function1/1(value), lbx_e/1, Mux1/1, Mux6/1
  Mux6/1 -> MATLAB Function2/1(value)
  Subsystem3/1(Out) -> Display5/1, Mux7/3, MATLAB Function5/1(value)
  Init2/1 -> MATLAB Function2/3(init_vector)
  Constant3/1 -> MATLAB Function2/2(length)
  MATLAB Function2/1(vector) -> Selector2/1
  Init1/1 -> MATLAB Function1/3(init_vector)
  Constant2/1 -> MATLAB Function1/2(length)
  MATLAB Function1/1(vector) -> Selector/1
  MATLAB Function/1(vector) -> Selector1/1
  Constant1/1 -> MATLAB Function/2(length)
  Init/1 -> MATLAB Function/3(init_vector)
  Mux4/1 -> Subsystem3/1(In)
  Mux2/1 -> Subsystem2/1(In)
  Mux5/1 -> Subsystem1/1(In)
  Mux/1 -> Subsystem/1(In)

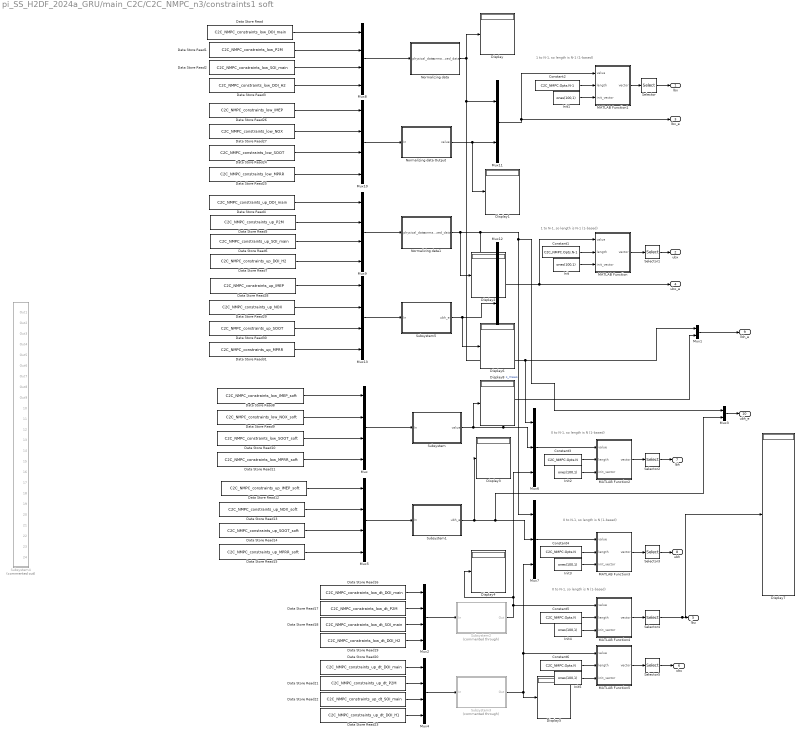
== system pi_SS_H2DF_2024a_GRU/main_C2C/C2C_NMPC_n3/constraints1 soft  ==
  note: 0 to N-1, so length is N (1-based)
  note: 0 to N-1, so length is N (1-based)
  note: 0 to N-1, so length is N (1-based)
  note: 1 to N-1, so length is N-1 (1-based)
  note: 1 to N-1, so length is N-1 (1-based)
  Constant1 : Constant  Value=C2C_NMPC.Opts.N-1
  Constant2 : Constant  Value=C2C_NMPC.Opts.N-1
  Constant{3..6} (4 alike) : Constant  Value=C2C_NMPC.Opts.N
  Data Store Read : DataStoreRead  DataStoreName=C2C_NMPC_constraints_low_DOI_main  IndexOptions=Index vector (dialog)  Indices=1  OutputSizes=1
  Data Store Read1 : DataStoreRead  DataStoreName=C2C_NMPC_constraints_low_P2M  IndexOptions=Index vector (dialog)  Indices=1  OutputSizes=1
  Data Store Read10 : DataStoreRead  DataStoreName=C2C_NMPC_constraints_low_SOOT_soft  IndexOptions=Index vector (dialog)  Indices=1  OutputSizes=1
  Data Store Read11 : DataStoreRead  DataStoreName=C2C_NMPC_constraints_low_MPRR_soft  IndexOptions=Index vector (dialog)  Indices=1  OutputSizes=1
  Data Store Read12 : DataStoreRead  DataStoreName=C2C_NMPC_constraints_up_IMEP_soft  IndexOptions=Index vector (dialog)  Indices=1  OutputSizes=1
  Data Store Read13 : DataStoreRead  DataStoreName=C2C_NMPC_constraints_up_NOX_soft  IndexOptions=Index vector (dialog)  Indices=1  OutputSizes=1
  Data Store Read14 : DataStoreRead  DataStoreName=C2C_NMPC_constraints_up_SOOT_soft  IndexOptions=Index vector (dialog)  Indices=1  OutputSizes=1
  Data Store Read15 : DataStoreRead  DataStoreName=C2C_NMPC_constraints_up_MPRR_soft  IndexOptions=Index vector (dialog)  Indices=1  OutputSizes=1
  Data Store Read16 : DataStoreRead  DataStoreName=C2C_NMPC_constraints_low_dt_DOI_main  IndexOptions=Index vector (dialog)  Indices=1  OutputSizes=1
  Data Store Read17 : DataStoreRead  DataStoreName=C2C_NMPC_constraints_low_dt_P2M  IndexOptions=Index vector (dialog)  Indices=1  OutputSizes=1
  Data Store Read18 : DataStoreRead  DataStoreName=C2C_NMPC_constraints_low_dt_SOI_main  IndexOptions=Index vector (dialog)  Indices=1  OutputSizes=1
  Data Store Read19 : DataStoreRead  DataStoreName=C2C_NMPC_constraints_low_dt_DOI_H2  IndexOptions=Index vector (dialog)  Indices=1  OutputSizes=1
  Data Store Read2 : DataStoreRead  DataStoreName=C2C_NMPC_constraints_low_SOI_main  IndexOptions=Index vector (dialog)  Indices=1  OutputSizes=1
  Data Store Read20 : DataStoreRead  DataStoreName=C2C_NMPC_constraints_up_dt_DOI_main  IndexOptions=Index vector (dialog)  Indices=1  OutputSizes=1
  Data Store Read21 : DataStoreRead  DataStoreName=C2C_NMPC_constraints_up_dt_P2M  IndexOptions=Index vector (dialog)  Indices=1  OutputSizes=1
  Data Store Read22 : DataStoreRead  DataStoreName=C2C_NMPC_constraints_up_dt_SOI_main  IndexOptions=Index vector (dialog)  Indices=1  OutputSizes=1
  Data Store Read23 : DataStoreRead  DataStoreName=C2C_NMPC_constraints_up_dt_DOI_H1  IndexOptions=Index vector (dialog)  Indices=1  OutputSizes=1
  Data Store Read24 : DataStoreRead  DataStoreName=C2C_NMPC_constraints_low_SOOT  IndexOptions=Index vector (dialog)  Indices=1  OutputSizes=1
  Data Store Read25 : DataStoreRead  DataStoreName=C2C_NMPC_constraints_low_MPRR  IndexOptions=Index vector (dialog)  Indices=1  OutputSizes=1
  Data Store Read26 : DataStoreRead  DataStoreName=C2C_NMPC_constraints_low_IMEP  IndexOptions=Index vector (dialog)  Indices=1  OutputSizes=1
  Data Store Read27 : DataStoreRead  DataStoreName=C2C_NMPC_constraints_low_NOX  IndexOptions=Index vector (dialog)  Indices=1  OutputSizes=1
  Data Store Read28 : DataStoreRead  DataStoreName=C2C_NMPC_constraints_up_IMEP  IndexOptions=Index vector (dialog)  Indices=1  OutputSizes=1
  Data Store Read29 : DataStoreRead  DataStoreName=C2C_NMPC_constraints_up_NOX  IndexOptions=Index vector (dialog)  Indices=1  OutputSizes=1
  Data Store Read3 : DataStoreRead  DataStoreName=C2C_NMPC_constraints_low_DOI_H2  IndexOptions=Index vector (dialog)  Indices=1  OutputSizes=1
  Data Store Read30 : DataStoreRead  DataStoreName=C2C_NMPC_constraints_up_SOOT  IndexOptions=Index vector (dialog)  Indices=1  OutputSizes=1
  Data Store Read31 : DataStoreRead  DataStoreName=C2C_NMPC_constraints_up_MPRR  IndexOptions=Index vector (dialog)  Indices=1  OutputSizes=1
  Data Store Read4 : DataStoreRead  DataStoreName=C2C_NMPC_constraints_up_DOI_main  IndexOptions=Index vector (dialog)  Indices=1  OutputSizes=1
  Data Store Read5 : DataStoreRead  DataStoreName=C2C_NMPC_constraints_up_P2M  IndexOptions=Index vector (dialog)  Indices=1  OutputSizes=1
  Data Store Read6 : DataStoreRead  DataStoreName=C2C_NMPC_constraints_up_SOI_main  IndexOptions=Index vector (dialog)  Indices=1  OutputSizes=1
  Data Store Read7 : DataStoreRead  DataStoreName=C2C_NMPC_constraints_up_DOI_H2  IndexOptions=Index vector (dialog)  Indices=1  OutputSizes=1
  Data Store Read8 : DataStoreRead  DataStoreName=C2C_NMPC_constraints_low_IMEP_soft  IndexOptions=Index vector (dialog)  Indices=1  OutputSizes=1
  Data Store Read9 : DataStoreRead  DataStoreName=C2C_NMPC_constraints_low_NOX_soft  IndexOptions=Index vector (dialog)  Indices=1  OutputSizes=1
  Display{,1..8} (9 alike) : Display
  Init{,1..5} (6 alike) : Constant  Value=ones(100,1)
  MATLAB Function : MATLAB Function  TreatAsAtomicUnit=on
  MATLAB Function1 : MATLAB Function  TreatAsAtomicUnit=on
  MATLAB Function2 : MATLAB Function  TreatAsAtomicUnit=on
  MATLAB Function3 : MATLAB Function  TreatAsAtomicUnit=on
  MATLAB Function4 : MATLAB Function  TreatAsAtomicUnit=on
  MATLAB Function5 : MATLAB Function  TreatAsAtomicUnit=on
  Mux{,2,4..5,8..10,13} (8 alike) : Mux
  Mux{1,3,11..12} (4 alike) : Mux  Inputs=2
  Mux6 : Mux  Inputs=3
  Mux7 : Mux  Inputs=3
  Normalizing data : Subsystem
  Normalizing data Output : Subsystem
  Normalizing data1 : Subsystem
  Selector : Selector  IndexOptions=Index vector (dialog)  Indices=1:((C2C_NMPC.Opts.N-1)*(C2C_NMPC.Dims.n_controls+C2C_NMPC.Dims.n_outputs))  OutputSizes=1
  Selector1 : Selector  IndexOptions=Index vector (dialog)  Indices=1:((C2C_NMPC.Opts.N-1)*(C2C_NMPC.Dims.n_controls+C2C_NMPC.Dims.n_outputs))  OutputSizes=1
  Selector2 : Selector  IndexOptions=Index vector (dialog)  Indices=1:((C2C_NMPC.Opts.N-1)*(C2C_NMPC.Dims.n_outputs + C2C_NMPC.Dims.n_controls +C2C_NMPC.Dims.n_controls))  OutputSizes=1
  Selector3 : Selector  IndexOptions=Index vector (dialog)  Indices=1:((C2C_NMPC.Opts.N-1)*(C2C_NMPC.Dims.n_outputs + C2C_NMPC.Dims.n_controls +C2C_NMPC.Dims.n_controls))  OutputSizes=1
  Selector4 : Selector  IndexOptions=Index vector (dialog)  Indices=1:((C2C_NMPC.Opts.N)*(C2C_NMPC.Dims.n_controls))  OutputSizes=1
  Selector5 : Selector  IndexOptions=Index vector (dialog)  Indices=1:((C2C_NMPC.Opts.N)*(C2C_NMPC.Dims.n_controls))  OutputSizes=1
  Subsystem : Subsystem
  Subsystem1 : Subsystem
  Subsystem2 : Subsystem  Commented=through
  Subsystem3 : Subsystem  Commented=through
  Subsystem4 : Subsystem  Commented=on
  Subsystem5 : Subsystem
  lbx : Outport
  ubx : Outport  Port=2
  lbx_e : Outport  Port=3
  ubx_e : Outport  Port=4
  lbu : Outport  Port=5
  ubu : Outport  Port=6
  lbh : Outport  Port=7
  ubh : Outport  Port=8
  lbh_e : Outport  Port=9
  ubh_e : Outport  Port=10
  wires:
  Mux/1 -> Subsystem/1(In)
  Mux5/1 -> Subsystem1/1(In)
  Mux2/1 -> Subsystem2/1(In)
  Mux4/1 -> Subsystem3/1(In)
  Init/1 -> MATLAB Function/3(init_vector)
  Constant1/1 -> MATLAB Function/2(length)
  MATLAB Function/1(vector) -> Selector1/1
  MATLAB Function1/1(vector) -> Selector/1
  Constant2/1 -> MATLAB Function1/2(length)
  Init1/1 -> MATLAB Function1/3(init_vector)
  MATLAB Function2/1(vector) -> Selector2/1
  Constant3/1 -> MATLAB Function2/2(length)
  Init2/1 -> MATLAB Function2/3(init_vector)
  Subsystem3/1(Out) -> MATLAB Function5/1(value), Mux7/3, Display5/1
  Mux6/1 -> MATLAB Function2/1(value)
  Normalizing data/1(normalized_data) -> Mux6/1, Mux1/1, Mux11/1, Display/1
  Subsystem/1(value) -> Display8/1, Mux1/2, Mux6/2
  Subsystem2/1(Out) -> MATLAB Function4/1(value), Display4/1, Mux6/3
  MATLAB Function3/1(vector) -> Selector3/1
  Mux7/1 -> MATLAB Function3/1(value)
  Init3/1 -> MATLAB Function3/3(init_vector)
  Constant4/1 -> MATLAB Function3/2(length)
  Data Store Read3/1 -> Mux8/4
  Data Store Read2/1 -> Mux8/3
  Data Store Read1/1 -> Mux8/2
  Data Store Read/1 -> Mux8/1
  Mux8/1 -> Normalizing data/1(physical_data)
  Selector/1 -> lbx/1
  Data Store Read6/1 -> Mux9/3
  Data Store Read5/1 -> Mux9/2
  Data Store Read4/1 -> Mux9/1
  Mux9/1 -> Normalizing data1/1(physical_data)
  Normalizing data1/1(normalized_data) -> Display2/1, Mux12/1, Mux7/1, Mux3/1  "x_meas"
  Data Store Read7/1 -> Mux9/4
  Selector1/1 -> ubx/1
  Selector2/1 -> lbh/1
  Selector3/1 -> ubh/1
  Mux1/1 -> lbh_e/1
  Subsystem1/1(ubh_e) -> Display3/1, Mux3/2, Mux7/2
  Mux3/1 -> ubh_e/1
  Data Store Read8/1 -> Mux/1
  Data Store Read9/1 -> Mux/2
  Data Store Read10/1 -> Mux/3
  Data Store Read11/1 -> Mux/4
  Data Store Read12/1 -> Mux5/1
  Data Store Read13/1 -> Mux5/2
  Data Store Read14/1 -> Mux5/3
  Data Store Read15/1 -> Mux5/4
  Data Store Read16/1 -> Mux2/1
  Data Store Read17/1 -> Mux2/2
  Data Store Read18/1 -> Mux2/3
  Data Store Read19/1 -> Mux2/4
  Data Store Read20/1 -> Mux4/1
  Data Store Read21/1 -> Mux4/2
  Data Store Read22/1 -> Mux4/3
  Data Store Read23/1 -> Mux4/4
  Constant5/1 -> MATLAB Function4/2(length)
  Init4/1 -> MATLAB Function4/3(init_vector)
  MATLAB Function4/1(vector) -> Selector4/1
  MATLAB Function5/1(vector) -> Selector5/1
  Init5/1 -> MATLAB Function5/3(init_vector)
  Constant6/1 -> MATLAB Function5/2(length)
  Selector5/1 -> ubu/1
  Selector4/1 -> Display7/1, lbu/1
  Data Store Read27/1 -> Mux10/2
  Data Store Read26/1 -> Mux10/1
  Data Store Read24/1 -> Mux10/3
  Data Store Read25/1 -> Mux10/4
  Mux10/1 -> Normalizing data Output/1(In)
  Mux11/1 -> lbx_e/1, MATLAB Function1/1(value)
  Normalizing data Output/1(value) -> Display1/1, Mux11/2
  Mux12/1 -> MATLAB Function/1(value), ubx_e/1
  Mux13/1 -> Subsystem5/1(In)
  Data Store Read30/1 -> Mux13/3
  Data Store Read29/1 -> Mux13/2
  Data Store Read28/1 -> Mux13/1
  Subsystem5/1(ubh_e) -> Display6/1, Mux12/2
  Data Store Read31/1 -> Mux13/4

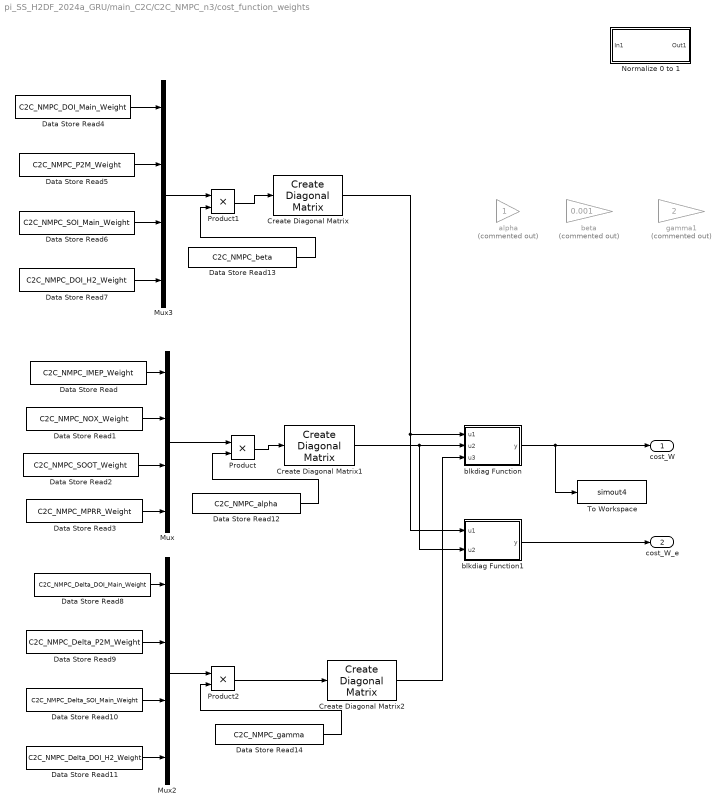
== system pi_SS_H2DF_2024a_GRU/main_C2C/C2C_NMPC_n3/cost_function_weights ==
  Create Diagonal Matrix : matrix_library/Create Diagonal Matrix
  Create Diagonal Matrix1 : matrix_library/Create Diagonal Matrix
  Create Diagonal Matrix2 : matrix_library/Create Diagonal Matrix
  Data Store Read : DataStoreRead  DataStoreName=C2C_NMPC_IMEP_Weight  IndexOptions=Index vector (dialog)  Indices=1  OutputSizes=1
  Data Store Read1 : DataStoreRead  DataStoreName=C2C_NMPC_NOX_Weight  IndexOptions=Index vector (dialog)  Indices=1  OutputSizes=1
  Data Store Read10 : DataStoreRead  DataStoreName=C2C_NMPC_Delta_SOI_Main_Weight  IndexOptions=Index vector (dialog)  Indices=1  OutputSizes=1
  Data Store Read11 : DataStoreRead  DataStoreName=C2C_NMPC_Delta_DOI_H2_Weight  IndexOptions=Index vector (dialog)  Indices=1  OutputSizes=1
  Data Store Read12 : DataStoreRead  DataStoreName=C2C_NMPC_alpha  IndexOptions=Index vector (dialog)  Indices=1  OutputSizes=1
  Data Store Read13 : DataStoreRead  DataStoreName=C2C_NMPC_beta  IndexOptions=Index vector (dialog)  Indices=1  OutputSizes=1
  Data Store Read14 : DataStoreRead  DataStoreName=C2C_NMPC_gamma  IndexOptions=Index vector (dialog)  Indices=1  OutputSizes=1
  Data Store Read2 : DataStoreRead  DataStoreName=C2C_NMPC_SOOT_Weight  IndexOptions=Index vector (dialog)  Indices=1  OutputSizes=1
  Data Store Read3 : DataStoreRead  DataStoreName=C2C_NMPC_MPRR_Weight  IndexOptions=Index vector (dialog)  Indices=1  OutputSizes=1
  Data Store Read4 : DataStoreRead  DataStoreName=C2C_NMPC_DOI_Main_Weight  IndexOptions=Index vector (dialog)  Indices=1  OutputSizes=1
  Data Store Read5 : DataStoreRead  DataStoreName=C2C_NMPC_P2M_Weight  IndexOptions=Index vector (dialog)  Indices=1  OutputSizes=1
  Data Store Read6 : DataStoreRead  DataStoreName=C2C_NMPC_SOI_Main_Weight  IndexOptions=Index vector (dialog)  Indices=1  OutputSizes=1
  Data Store Read7 : DataStoreRead  DataStoreName=C2C_NMPC_DOI_H2_Weight  IndexOptions=Index vector (dialog)  Indices=1  OutputSizes=1
  Data Store Read8 : DataStoreRead  DataStoreName=C2C_NMPC_Delta_DOI_Main_Weight  IndexOptions=Index vector (dialog)  Indices=1  OutputSizes=1
  Data Store Read9 : DataStoreRead  DataStoreName=C2C_NMPC_Delta_P2M_Weight  IndexOptions=Index vector (dialog)  Indices=1  OutputSizes=1
  Mux : Mux
  Mux2 : Mux
  Mux3 : Mux
  Normalize 0 to 1 : Subsystem
  Product : Product
  Product1 : Product
  Product2 : Product
  To Workspace : ToWorkspace  VariableName=simout4  SaveFormat=Timeseries  SampleTime=-1
  alpha : Gain  Commented=on
  beta : Gain  Commented=on  Gain=0.001
  blkdiag Function : MATLAB Function  TreatAsAtomicUnit=on
  blkdiag Function1 : MATLAB Function  TreatAsAtomicUnit=on
  gamma1 : Gain  Commented=on  Gain=2
  cost_W : Outport
  cost_W_e : Outport  Port=2
  wires:
  blkdiag Function1/1(y) -> cost_W_e/1
  Mux2/1 -> Product2/1
  Data Store Read14/1 -> Product2/2
  Data Store Read13/1 -> Product1/2
  Data Store Read12/1 -> Product/2
  Data Store Read11/1 -> Mux2/4
  Data Store Read10/1 -> Mux2/3
  Data Store Read9/1 -> Mux2/2
  Data Store Read8/1 -> Mux2/1
  Create Diagonal Matrix/1 -> blkdiag Function/1(u1), blkdiag Function1/1(u1)
  Data Store Read2/1 -> Mux/3
  Data Store Read3/1 -> Mux/4
  Data Store Read/1 -> Mux/1
  Data Store Read1/1 -> Mux/2
  Mux/1 -> Product/1
  Product/1 -> Create Diagonal Matrix1/1
  Product1/1 -> Create Diagonal Matrix/1
  Mux3/1 -> Product1/1
  Data Store Read5/1 -> Mux3/2
  Data Store Read6/1 -> Mux3/3
  Data Store Read4/1 -> Mux3/1
  Data Store Read7/1 -> Mux3/4
  Create Diagonal Matrix1/1 -> blkdiag Function/2(u2), blkdiag Function1/2(u2)
  Product2/1 -> Create Diagonal Matrix2/1
  Create Diagonal Matrix2/1 -> blkdiag Function/3(u3)
  blkdiag Function/1(y) -> cost_W/1, To Workspace/1
